simulink model "ED3"  (R2014a)
settings: Solver=ode45  StartTime=0.0  StopTime=100  RelTol=1e-3
undefined symbols (not defined in the file): Kd, Ki, Kp
settings Model: Creator=Fabia  LastModifiedBy=Fabia

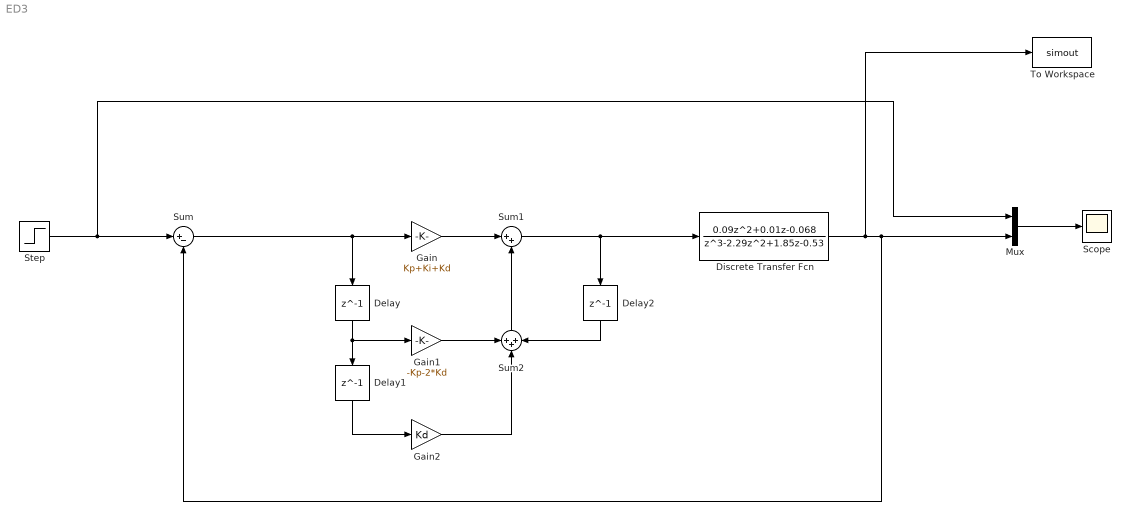
== system ED3 ==
  Delay : Delay  DelayLength=1  InitialCondition=0
  Delay1 : Delay  DelayLength=1  InitialCondition=0
  Delay2 : Delay  DelayLength=1  InitialCondition=0
  Discrete Transfer Fcn : DiscreteTransferFcn  Numerator=[0.09 0.01 -0.068]  Denominator=[1 -2.29 1.85 -0.53]
  Gain : Gain  Gain=Kp+Ki+Kd
  Gain1 : Gain  Gain=-Kp-2*Kd
  Gain2 : Gain  Gain=Kd
  Mux : Mux  Inputs=2
  Scope : Scope
  Step : Step  Time=0  SampleTime=1
  Sum : Sum  Inputs=|+-
  Sum1 : Sum  Inputs=|++
  Sum2 : Sum  Inputs=+++
  To Workspace : ToWorkspace  VariableName=simout  SampleTime=-1
  wires:
  Step/1 -> Mux/1, Sum/1
  Discrete Transfer Fcn/1 -> To Workspace/1, Sum/2, Mux/2
  Mux/1 -> Scope/1
  Sum/1 -> Gain/1, Delay/1
  Delay/1 -> Gain1/1, Delay1/1
  Delay1/1 -> Gain2/1
  Gain/1 -> Sum1/1
  Sum1/1 -> Delay2/1, Discrete Transfer Fcn/1
  Sum2/1 -> Sum1/2
  Gain1/1 -> Sum2/1
  Delay2/1 -> Sum2/3
  Gain2/1 -> Sum2/2
